simulink model "joystick_receiveUDPpacket"  (R2024a)
settings: Solver=FixedStepAuto  StartTime=0.0  StopTime=inf  RelTol=1e-3
libraries: slrealtimeutilitieslib x7, slrealtimeiplib x2
settings Model: Creator=matlab.cut  LastModifiedBy=matlab.cut
settings SolverCC: ConcurrentTasks=on  PositivePriorityOrder=on
settings OptimizationCC: BlockReduction=off  OptimizeBlockIOStorage=off
settings DebuggingCC: TasksWithSamePriorityMsg=none
settings HardwareCC: ProdBitPerLong=64  ProdLongLongMode=on  ProdHWDeviceType=Intel->x86-64 (Linux 64)
settings RTWCC: Description=Speedgoat Real-Time Target Machine  SystemTargetFile=speedgoat.tlc  TemplateMakefile=slrealtime_default_tmf  Toolchain=Simulink Real-Time Toolchain  BuildConfiguration=Faster Runs  CodeExecutionProfiling=on  TargetLang=C++
settings SimulinkRealTimeTargetCC: InstructionSetFMA=off  LogToMDFFile=off

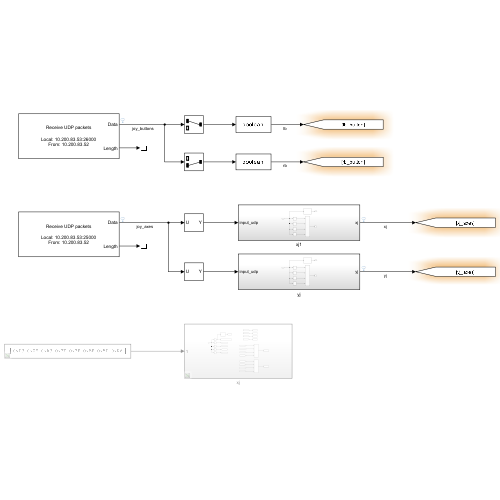
[thumbnail: Simulink's stored preview of the top-level diagram]
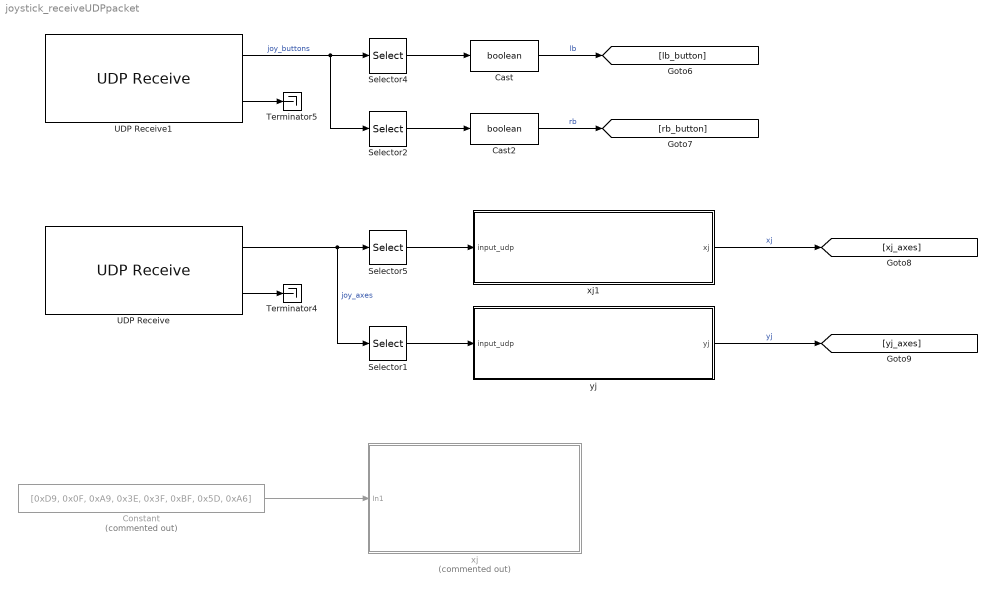
== system joystick_receiveUDPpacket ==
  Cast : DataTypeConversion  OutDataTypeStr=boolean  SaturateOnIntegerOverflow=off  RndMeth=Floor
  Cast2 : DataTypeConversion  OutDataTypeStr=boolean  SaturateOnIntegerOverflow=off  RndMeth=Floor
  Constant : Constant  Commented=on  Value=[0xD9, 0x0F, 0xA9, 0x3E, 0x3F, 0xBF, 0x5D, 0xA6]
  Selector1 : Selector  InputPortWidth=8  IndexOptions=Index vector (dialog)  Indices=[5:8]  OutputSizes=1
  Selector2 : Selector  InputPortWidth=2  IndexOptions=Index vector (dialog)  Indices=2  OutputSizes=1
  Selector4 : Selector  InputPortWidth=2  IndexOptions=Index vector (dialog)  Indices=1  OutputSizes=1
  Selector5 : Selector  InputPortWidth=8  IndexOptions=Index vector (dialog)  Indices=[1:4]  OutputSizes=1
  Terminator4 : Terminator
  Terminator5 : Terminator
  UDP Receive : slrealtimeiplib/UDP Receive  useHostTargetConn=off  ipAddress=10.200.83.53  localPort=25000  rcvWidth=8  rcvFmAny=off  fmAddress='10.200.83.52'  sampleTime=1e-3  enableMessage=off  maxPackets=1
  UDP Receive1 : slrealtimeiplib/UDP Receive  useHostTargetConn=off  ipAddress=10.200.83.53  localPort=26000  rcvWidth=2  rcvFmAny=off  fmAddress='10.200.83.52'  sampleTime=1e-3  enableMessage=off  maxPackets=1
  xj : Subsystem  Commented=on
  xj1 : Subsystem
  yj : Subsystem
  wires:
  Constant/1 -> xj/1(In1)
  Cast/1 -> [lb_button]  "lb"
  Cast2/1 -> [rb_button]  "rb"
  Selector4/1 -> Cast/1
  Selector5/1 -> xj1/1(input_udp)
  UDP Receive1/2 -> Terminator5/1
  xj1/1(xj) -> [xj_axes]  "xj"
  UDP Receive1/1 -> Selector4/1, Selector2/1  "joy_buttons"
  Selector1/1 -> yj/1(input_udp)
  Selector2/1 -> Cast2/1
  UDP Receive/1 -> Selector5/1, Selector1/1  "joy_axes"
  UDP Receive/2 -> Terminator4/1
  yj/1(yj) -> [yj_axes]  "yj"

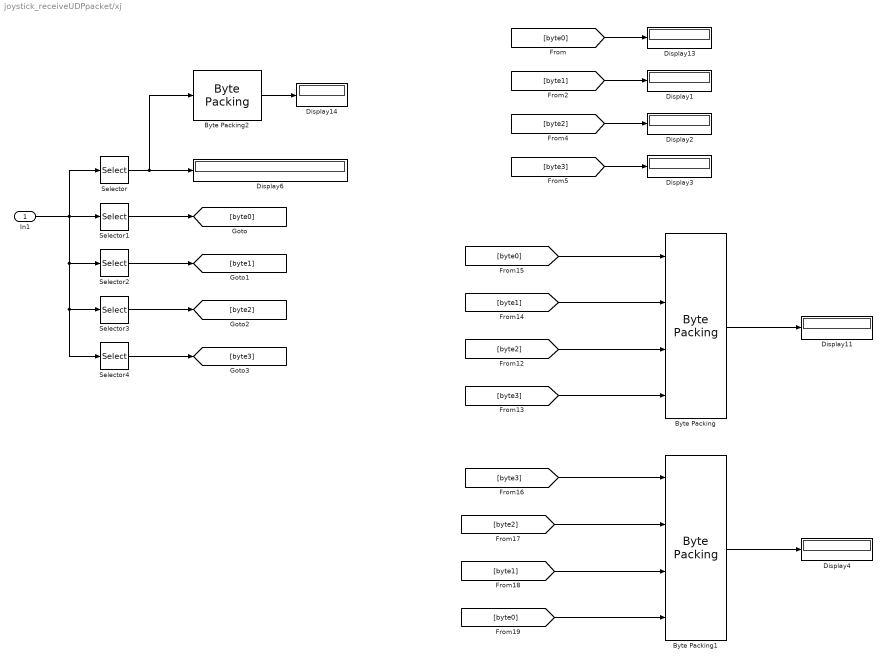
== system joystick_receiveUDPpacket/xj ==
  In1 : Inport
  Byte Packing : slrealtimeutilitieslib/Byte Packing  MaskPackedDataType=single  MaskUnpackedDataTypes={'uint8','uint8','uint8','uint8'}  MaskAlignment=1
  Byte Packing1 : slrealtimeutilitieslib/Byte Packing  MaskPackedDataType=single  MaskUnpackedDataTypes={'uint8','uint8','uint8','uint8'}  MaskAlignment=1
  Byte Packing2 : slrealtimeutilitieslib/Byte Packing  MaskPackedDataType=single  MaskUnpackedDataTypes={'uint8'}  MaskAlignment=1
  Display{1..4,6,11,13..14} (8 alike) : Display
      Display1 settings: Format=hex (Stored Integer)
      Display13 settings: Format=hex (Stored Integer)
      Display2 settings: Format=hex (Stored Integer)
      Display3 settings: Format=hex (Stored Integer)
      Display6 settings: Format=hex (Stored Integer)
  Selector : Selector  InputPortWidth=8  IndexOptions=Index vector (dialog)  Indices=[1:4]  OutputSizes=1
  Selector1 : Selector  InputPortWidth=8  IndexOptions=Index vector (dialog)  Indices=1  OutputSizes=1
  Selector2 : Selector  InputPortWidth=8  IndexOptions=Index vector (dialog)  Indices=2  OutputSizes=1
  Selector3 : Selector  InputPortWidth=8  IndexOptions=Index vector (dialog)  Indices=3  OutputSizes=1
  Selector4 : Selector  InputPortWidth=8  IndexOptions=Index vector (dialog)  Indices=4  OutputSizes=1
  wires:
  In1/1 -> Selector1/1, Selector/1, Selector2/1, Selector4/1, Selector3/1
  Selector1/1 -> [byte0]
  Selector2/1 -> [byte1]
  Selector3/1 -> [byte2]
  Selector4/1 -> [byte3]
  [byte0] -> Display13/1
  [byte2] -> Display2/1
  [byte1] -> Display1/1
  [byte3] -> Display3/1
  Selector/1 -> Byte Packing2/1, Display6/1
  [byte0] -> Byte Packing/1
  [byte1] -> Byte Packing/2
  [byte2] -> Byte Packing/3
  [byte3] -> Byte Packing/4
  Byte Packing/1 -> Display11/1
  Byte Packing1/1 -> Display4/1
  [byte0] -> Byte Packing1/4
  [byte1] -> Byte Packing1/3
  [byte2] -> Byte Packing1/2
  [byte3] -> Byte Packing1/1
  Byte Packing2/1 -> Display14/1

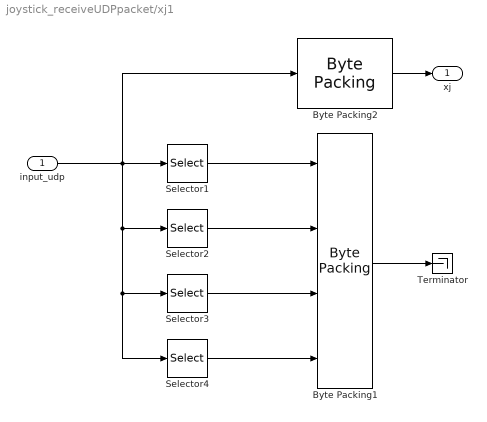
== system joystick_receiveUDPpacket/xj1 ==
  input_udp : Inport
  Byte Packing1 : slrealtimeutilitieslib/Byte Packing  MaskPackedDataType=single  MaskUnpackedDataTypes={'uint8','uint8','uint8','uint8'}  MaskAlignment=1
  Byte Packing2 : slrealtimeutilitieslib/Byte Packing  MaskPackedDataType=single  MaskUnpackedDataTypes={'uint8'}  MaskAlignment=1
  Selector1 : Selector  InputPortWidth=4  IndexOptions=Index vector (dialog)  Indices=1  OutputSizes=1
  Selector2 : Selector  InputPortWidth=4  IndexOptions=Index vector (dialog)  Indices=2  OutputSizes=1
  Selector3 : Selector  InputPortWidth=4  IndexOptions=Index vector (dialog)  Indices=3  OutputSizes=1
  Selector4 : Selector  InputPortWidth=4  IndexOptions=Index vector (dialog)  Indices=4  OutputSizes=1
  Terminator : Terminator
  xj : Outport
  wires:
  Byte Packing1/1 -> Terminator/1
  Byte Packing2/1 -> xj/1
  Selector1/1 -> Byte Packing1/1
  Selector2/1 -> Byte Packing1/2
  input_udp/1 -> Byte Packing2/1, Selector4/1, Selector3/1, Selector2/1, Selector1/1
  Selector3/1 -> Byte Packing1/3
  Selector4/1 -> Byte Packing1/4

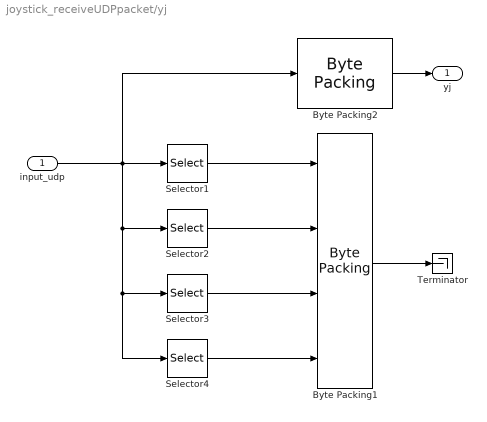
== system joystick_receiveUDPpacket/yj ==
  input_udp : Inport
  Byte Packing1 : slrealtimeutilitieslib/Byte Packing  MaskPackedDataType=single  MaskUnpackedDataTypes={'uint8','uint8','uint8','uint8'}  MaskAlignment=1
  Byte Packing2 : slrealtimeutilitieslib/Byte Packing  MaskPackedDataType=single  MaskUnpackedDataTypes={'uint8'}  MaskAlignment=1
  Selector1 : Selector  InputPortWidth=4  IndexOptions=Index vector (dialog)  Indices=1  OutputSizes=1
  Selector2 : Selector  InputPortWidth=4  IndexOptions=Index vector (dialog)  Indices=2  OutputSizes=1
  Selector3 : Selector  InputPortWidth=4  IndexOptions=Index vector (dialog)  Indices=3  OutputSizes=1
  Selector4 : Selector  InputPortWidth=4  IndexOptions=Index vector (dialog)  Indices=4  OutputSizes=1
  Terminator : Terminator
  yj : Outport
  wires:
  Byte Packing1/1 -> Terminator/1
  Byte Packing2/1 -> yj/1
  Selector1/1 -> Byte Packing1/1
  Selector2/1 -> Byte Packing1/2
  input_udp/1 -> Byte Packing2/1, Selector4/1, Selector3/1, Selector2/1, Selector1/1
  Selector3/1 -> Byte Packing1/3
  Selector4/1 -> Byte Packing1/4
